simulink model "STM32_Nucleo_DataDumping"  (R2023a)
settings: Solver=FixedStepAuto  StartTime=0.0  StopTime=inf  FixedStep=0.001  RelTol=1e-3
libraries: stmutilitieslib x10, instrumentseriallib x2, mspfiltlib x1
settings Model: Creator=JesseJabezArendse  LastModifiedBy=JesseJabezArendse
settings DebuggingCC: ParameterPrecisionLossMsg=none

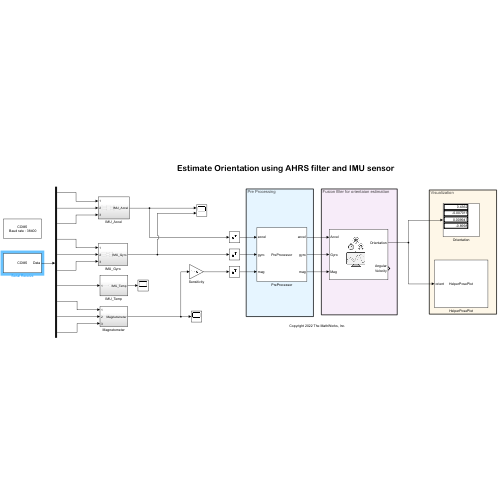
[thumbnail: Simulink's stored preview of the top-level diagram]
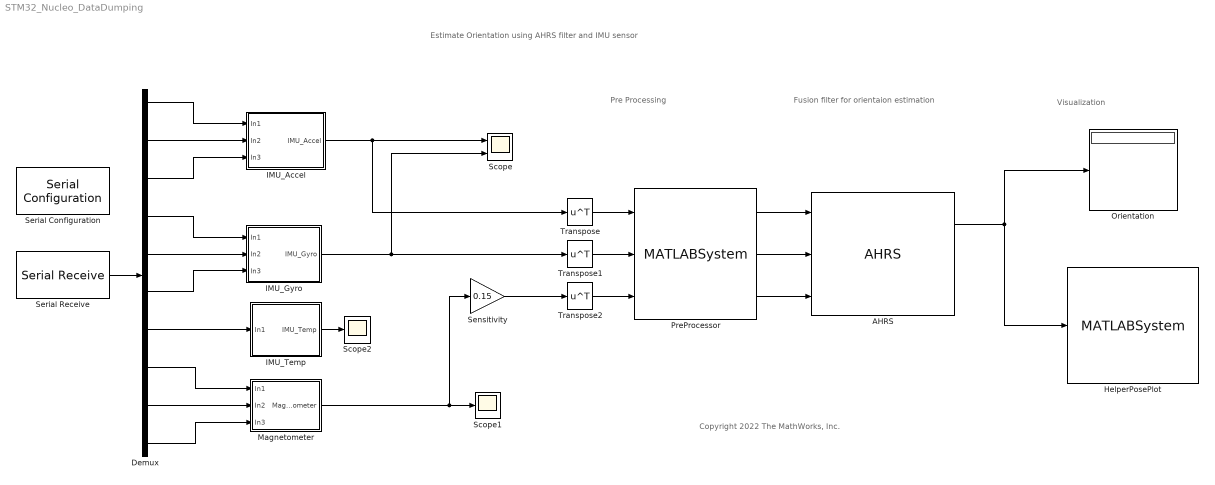
== system STM32_Nucleo_DataDumping ==
  note: Estimate Orientation using AHRS filter and IMU sensor
  note: Visualization
  note: Fusion filter for orientaion estimation
  note: Copyright 2022 The MathWorks, Inc.
  note: Pre Processing
  AHRS : mspfiltlib/AHRS  DispRefFrame=NED  DecimationFactor=1  InitialProcessNoise=ahrsfilter.defaultProcessNoise  OrientationFormat=quaternion  SimulateUsing=Code generation  AccelerometerNoise=0.0001924722  GyroscopeNoise=9.1385e-5  MagnetometerNoise=0.1  GyroscopeDriftNoise=12.0462e-13  LinearAccelerationNoise=0.0096236100000000012  MagneticDisturbanceNoise=0.5  LinearAccelerationDecayFactor=0.5  MagneticDisturbanceDecayFactor=0.5  ExpectedMagneticFieldStrength=50
  Demux : Demux  Outputs=[8 8 8 8 8 8 8 2 2 2]
  HelperPosePlot : MATLABSystem  System=HelperPosePlot  OrientationFormat=Quaternion
      mask Type: HelperPosePlot
      mask Display:
      | disp('HelperPosePlot');
      | port_label('input',1,'orient');
  IMU_Accel : Subsystem
  IMU_Gyro : Subsystem
  IMU_Temp : Subsystem
  Magnetometer : Subsystem
  Orientation : Display
  PreProcessor : MATLABSystem  System=PreProcessor  MagOffsets=[0,0,0]  AccelXAxisIndex=1  AccelXAxisSign=+  AccelYAxisIndex=2  AccelYAxisSign=+  AccelZAxisIndex=3  AccelZAxisSign=+  GyroXAxisIndex=1  GyroXAxisSign=+  GyroYAxisIndex=2  GyroYAxisSign=+  GyroZAxisIndex=3  GyroZAxisSign=+  MagXAxisIndex=1  MagXAxisSign=+  MagYAxisIndex=2  MagYAxisSign=-  MagZAxisIndex=3  MagZAxisSign=+
      mask Type: PreProcessor
      mask Display:
      | disp('PreProcessor');
      | port_label('input',1,'accel');
      | port_label('input',2,'gyro');
      | port_label('input',3,'mag');
      | port_label('output',1,'accel');
      | port_label('output',2,'gyro');
      | port_label('output',3,'mag');
  Scope : Scope  NumInputPorts=2
  Scope1 : Scope
  Scope2 : Scope
  Sensitivity : Gain  Gain=0.15  OutDataTypeStr=double  LockScale=on
  Serial Configuration : instrumentseriallib/Serial Configuration  Priority=-200000  PortSel=COM5  Port=COM5  ComPort=COM5  BaudRate=38400  DataBits=8  Parity=none  StopBits=1  ByteOrder=little-endian  FlowControl=none  Timeout=10  SimulateUsing=Interpreted execution  BlockInModel=on  aMode=1
      settings: LibrarySourceBlock=embeddedtargetslib/Host Communication/Serial Configuration
  Serial Receive : instrumentseriallib/Serial Receive  Priority=1  PortSel=COM5  Port=COM5  ComPort=COM5  DataType=uint8  SaveDataType=uint8  ToggleHeader=on  Header='JJA'  ToggleTerminator=on  Terminator=Custom terminator  CustomTerminator='AP_1'  InputFormat=Column major  ToggleDataSize=on  DataSize=[1 62]  EnableBlockingMode=on  ActionDataUnavailable=Output last received value  ActionWhenDataUnavailable=Output last received value  CustomValue=0  SampleTime=0.2  SimulateUsing=Interpreted execution  BlockInModel=on  aMode=1
      settings: LibrarySourceBlock=embeddedtargetslib/Host Communication/Serial Receive
  Transpose : Math  Operator=transpose
  Transpose1 : Math  Operator=transpose
  Transpose2 : Math  Operator=transpose
  wires:
  Serial Receive/1 -> Demux/1
  Demux/1 -> IMU_Accel/1(In1)
  Demux/2 -> IMU_Accel/2(In2)
  Demux/3 -> IMU_Accel/3(In3)
  Demux/4 -> IMU_Gyro/1(In1)
  Demux/5 -> IMU_Gyro/2(In2)
  Demux/6 -> IMU_Gyro/3(In3)
  Demux/8 -> Magnetometer/1(In1)
  Demux/9 -> Magnetometer/2(In2)
  Demux/7 -> IMU_Temp/1(In1)
  AHRS/1 -> Orientation/1, HelperPosePlot/1
  PreProcessor/1 -> AHRS/1
  PreProcessor/3 -> AHRS/3
  PreProcessor/2 -> AHRS/2
  Demux/10 -> Magnetometer/3(In3)
  Magnetometer/1(Magnetometer) -> Sensitivity/1, Scope1/1
  Sensitivity/1 -> Transpose2/1
  IMU_Accel/1(IMU_Accel) -> Transpose/1, Scope/1
  IMU_Gyro/1(IMU_Gyro) -> Transpose1/1, Scope/2
  Transpose/1 -> PreProcessor/1
  Transpose1/1 -> PreProcessor/2
  Transpose2/1 -> PreProcessor/3
  IMU_Temp/1(IMU_Temp) -> Scope2/1

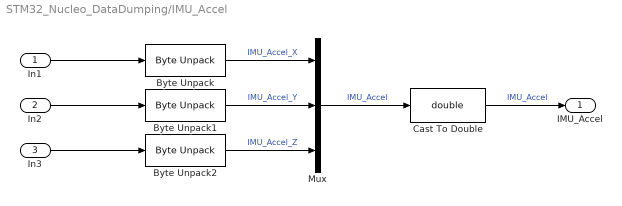
== system STM32_Nucleo_DataDumping/IMU_Accel ==
  In1 : Inport
  In2 : Inport  Port=2
  In3 : Inport  Port=3
  Byte Unpack : stmutilitieslib/Byte Unpack  dimensions={[1]}  datatypes={'double'}  byteAlign=1  blockPlatform=stm32f4discovery
  Byte Unpack1 : stmutilitieslib/Byte Unpack  dimensions={[1]}  datatypes={'double'}  byteAlign=1  blockPlatform=stm32f4discovery
  Byte Unpack2 : stmutilitieslib/Byte Unpack  dimensions={[1]}  datatypes={'double'}  byteAlign=1  blockPlatform=stm32f4discovery
  Cast To Double : DataTypeConversion  OutDataTypeStr=double  SaturateOnIntegerOverflow=off  RndMeth=Floor
  Mux : Mux  Inputs=3
  IMU_Accel : Outport
  wires:
  Byte Unpack/1 -> Mux/1  "IMU_Accel_X"
  Byte Unpack2/1 -> Mux/3  "IMU_Accel_Z"
  In2/1 -> Byte Unpack1/1
  Byte Unpack1/1 -> Mux/2  "IMU_Accel_Y"
  In1/1 -> Byte Unpack/1
  Cast To Double/1 -> IMU_Accel/1  "IMU_Accel"
  In3/1 -> Byte Unpack2/1
  Mux/1 -> Cast To Double/1  "IMU_Accel"

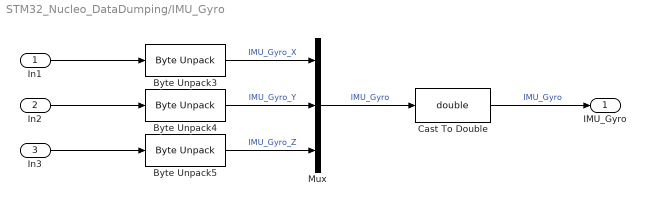
== system STM32_Nucleo_DataDumping/IMU_Gyro ==
  In1 : Inport
  In2 : Inport  Port=2
  In3 : Inport  Port=3
  Byte Unpack3 : stmutilitieslib/Byte Unpack  dimensions={[1]}  datatypes={'double'}  byteAlign=1  blockPlatform=stm32f4discovery
  Byte Unpack4 : stmutilitieslib/Byte Unpack  dimensions={[1]}  datatypes={'double'}  byteAlign=1  blockPlatform=stm32f4discovery
  Byte Unpack5 : stmutilitieslib/Byte Unpack  dimensions={[1]}  datatypes={'double'}  byteAlign=1  blockPlatform=stm32f4discovery
  Cast To Double : DataTypeConversion  OutDataTypeStr=double  SaturateOnIntegerOverflow=off  RndMeth=Floor
  Mux : Mux  Inputs=3
  IMU_Gyro : Outport
  wires:
  Cast To Double/1 -> IMU_Gyro/1  "IMU_Gyro"
  Byte Unpack5/1 -> Mux/3  "IMU_Gyro_Z"
  Byte Unpack3/1 -> Mux/1  "IMU_Gyro_X"
  In2/1 -> Byte Unpack4/1
  In1/1 -> Byte Unpack3/1
  Byte Unpack4/1 -> Mux/2  "IMU_Gyro_Y"
  In3/1 -> Byte Unpack5/1
  Mux/1 -> Cast To Double/1  "IMU_Gyro"

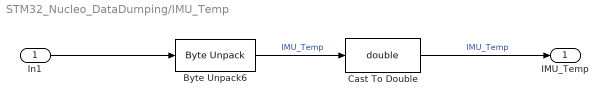
== system STM32_Nucleo_DataDumping/IMU_Temp ==
  In1 : Inport
  Byte Unpack6 : stmutilitieslib/Byte Unpack  dimensions={[1]}  datatypes={'double'}  byteAlign=1  blockPlatform=stm32f4discovery
  Cast To Double : DataTypeConversion  OutDataTypeStr=double  SaturateOnIntegerOverflow=off  RndMeth=Floor
  IMU_Temp : Outport
  wires:
  In1/1 -> Byte Unpack6/1
  Cast To Double/1 -> IMU_Temp/1  "IMU_Temp"
  Byte Unpack6/1 -> Cast To Double/1  "IMU_Temp"

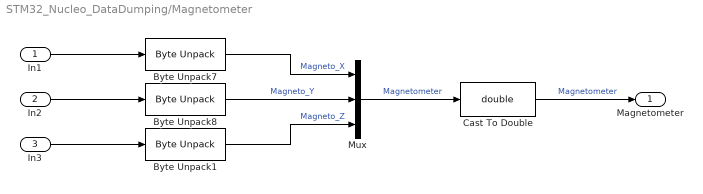
== system STM32_Nucleo_DataDumping/Magnetometer ==
  In1 : Inport
  In2 : Inport  Port=2
  In3 : Inport  Port=3
  Byte Unpack1 : stmutilitieslib/Byte Unpack  dimensions={[1]}  datatypes={'int16'}  byteAlign=1  blockPlatform=stm32f4discovery
  Byte Unpack7 : stmutilitieslib/Byte Unpack  dimensions={[1]}  datatypes={'int16'}  byteAlign=1  blockPlatform=stm32f4discovery
  Byte Unpack8 : stmutilitieslib/Byte Unpack  dimensions={[1]}  datatypes={'int16'}  byteAlign=1  blockPlatform=stm32f4discovery
  Cast To Double : DataTypeConversion  OutDataTypeStr=double  SaturateOnIntegerOverflow=off  RndMeth=Floor
  Mux : Mux  Inputs=3
  Magnetometer : Outport
  wires:
  Byte Unpack7/1 -> Mux/1  "Magneto_X"
  Cast To Double/1 -> Magnetometer/1  "Magnetometer"
  In1/1 -> Byte Unpack7/1
  Byte Unpack8/1 -> Mux/2  "Magneto_Y"
  In2/1 -> Byte Unpack8/1
  In3/1 -> Byte Unpack1/1
  Byte Unpack1/1 -> Mux/3  "Magneto_Z"
  Mux/1 -> Cast To Double/1  "Magnetometer"
